simulink model "WiperSystemStateflow"  (R2022b)
settings: Solver=FixedStepDiscrete  StartTime=0.0  StopTime=20  FixedStep=0.01  RelTol=1e-3
undefined symbols (not defined in the file): sigbuilder_block
libraries: eeGeneralControl x1
settings Model: Creator=AymanLaptop  LastModifiedBy=AymanLaptop

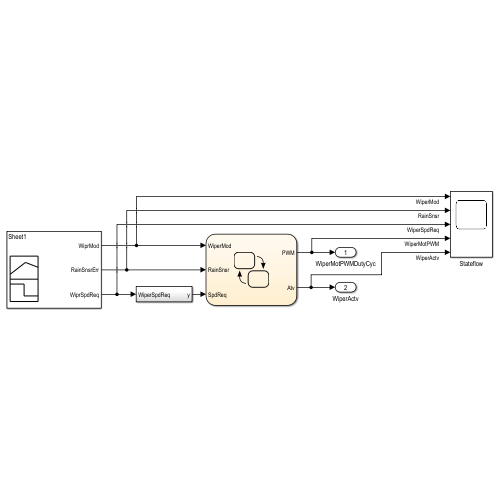
[thumbnail: Simulink's stored preview of the top-level diagram]
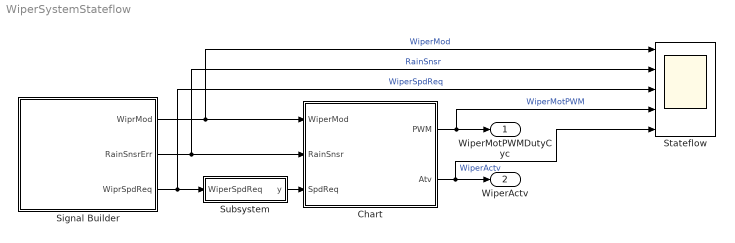
== system WiperSystemStateflow ==
  Chart : Stateflow chart  TreatAsAtomicUnit=on
      settings: PortSchema="{\"entries\":[{\"content\":{\"sides\":[{\"content\":{\"connectorIds\":[\"In2\",\"In1\",\"In3\"]},\"type\":\"ConnectorPlacement.EquallySpacedRectSide\",\"uuid\":\"e733ae65-f33e-49b0-845d-2dd686951ef3\"},{\"content\":{\"connectorIds\":[\"Out1\",\"Out2\"],\"side\":\"RIGHT\"},\"type\":\"ConnectorPlacement.EquallySpacedRectSide\",\"uuid\":\"70e09a91-b04b-4e75-a97f-4ab4b2922f79\"},{\"content\":{\"connectorIds\":[],\"side\":\"TOP\"},\"type\":\"ConnectorPlacement.EquallySpacedRectSide\",\"uuid\":\"7af5aa97-ae43-4f6a-8202-2e08a2f2b9b4\"}]},\"type\":\"ConnectorPlacement.EquallySpacedConnector\",\"uuid\":\"991bf9ea-0f6f-4566-8b19-b62aabc6abff\"}],\"packageUris\":[\"http://schema.mathworks.com/mf0/Connector/R2020b\"],\"version\":\"1.0\"}"
  Signal Builder : Subsystem  Tag=STV Subsys  LoadFcn=sigbuilder_block('load');  StartFcn=sigbuilder_block('start');  StopFcn=sigbuilder_block('stop');  ClipboardFcn=sigbuilder_block('clipboard');  mask(Sigbuilder block){tuvar=[0:10]}
      mask help: Simulink:masks:SigbuilderBlock_MD
      mask init:
      | if ~strcmp(get_param(bdroot(gcbh),'SimulationStatus'),'stopped') tuvar = sigbuilder_block('maskInit'); end
      settings: CopyFcn=sigbuilder_block('copy');  DeleteFcn=sigbuilder_block('delete');  ModelCloseFcn=sigbuilder_block('modelClose');  PreSaveFcn=sigbuilder_block('preSave');  PauseFcn=sigbuilder_block('pause');  ContinueFcn=sigbuilder_block('continue');  NameChangeFcn=sigbuilder_block('namechange');  OpenFcn=sigbuilder_block('open',[6 0 1012.5 455.25 ]);  CloseFcn=sigbuilder_block('close');
      mask Display: plot(0, 0, 100, 100,[2, 2, 32, 32, 2], [68, 8, 8, 68, 68],[32, 2], [38, 38], [32, 19, 2],[53, 60, 44], [32, 17, 17, 2],[16, 16, 31, 31]);txt = getActiveGroup(gcbh);text(2, 100, txt,'verticalAlignment', 'top');
  Stateflow : Scope  NumInputPorts=5
  Subsystem : Subsystem
  WiperMotPWMDutyCyc : Outport
  WiperActv : Outport  Port=2
  wires:
  Chart/2(Atv) -> WiperActv/1, Stateflow/5  "WiperActv"
  Signal Builder/1(WiprMod) -> Chart/2(WiperMod), Stateflow/1  "WiperMod"
  Signal Builder/3(WiprSpdReq) -> Stateflow/3, Subsystem/1(WiperSpdReq)  "WiperSpdReq"
  Signal Builder/2(RainSnsrErr) -> Chart/1(RainSnsr), Stateflow/2  "RainSnsr"
  Chart/1(PWM) -> WiperMotPWMDutyCyc/1, Stateflow/4  "WiperMotPWM"
  Subsystem/1(y) -> Chart/3(SpdReq)

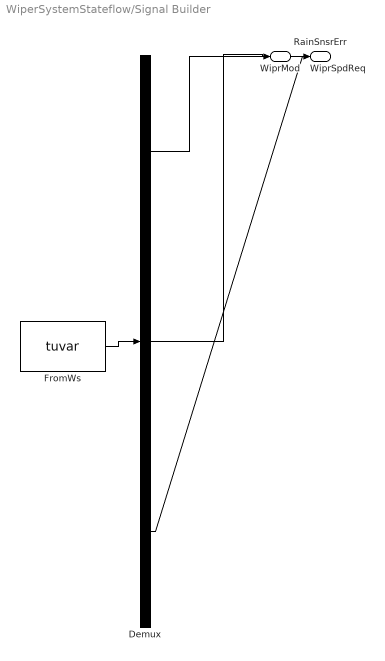
== system WiperSystemStateflow/Signal Builder ==
  Demux : Demux  Tag=STV Demux  Outputs=3
      settings: DisplayOption=none
  FromWs : FromWorkspace  Tag=STV FromWs  VariableName=tuvar  SampleTime=1  OutputAfterFinalValue=Holding final value
      SigBuilderData=|
      | common.afterFinalStr = 'Hold final value'
      | common.sampleTime = '1'
      | dataSet.timeRange = [0 16]
      | dataSet.name = 'Sheet1'
      | sbobj.Groups.Name = 'Sheet1'
      | sbobj.Groups.Signals(1).Name = 'WiprMod'
      | sbobj.Groups.Signals(1).XData = [0 1 2 3 4 5 6 7 8 9 10 11 12 13 14 15 16]
      | sbobj.Groups.Signals(1).YData = [0 0 2 2 3 3 1 1 1 1 1 1 1 1 1 1 1]
      | sbobj.Groups.Signals(2).Name = 'RainSnsrErr'
      | sbobj.Groups.Signals(2).XData = [0 1 2 3 4 5 6 7 8 9 10 11 12 13 14 15 16]
      | sbobj.Groups.Signals(2).YData = [0 0 0 0 0 0 0 0 0 0 0 0 0 0 0 1 0]
      | sbobj.Groups.Signals(3).Name = 'WiprSpdReq'
      | sbobj.Groups.Signals(3).XData = [0 1 2 3 4 5 6 7 8 9 10 11 12 13 14 15 16]
      | sbobj.Groups.Signals(3).YData = [0 0 0 0 0 0 0 0 1 2 3 4 5 6 7 7 7]
      | sbobj.Groups.TimeRange = [0 16]
  WiprMod : Outport  Tag=STV Outport
  RainSnsrErr : Outport  Tag=STV Outport  Port=2
  WiprSpdReq : Outport  Tag=STV Outport  Port=3
  wires:
  Demux/1 -> WiprMod/1
  FromWs/1 -> Demux/1
  Demux/2 -> RainSnsrErr/1
  Demux/3 -> WiprSpdReq/1

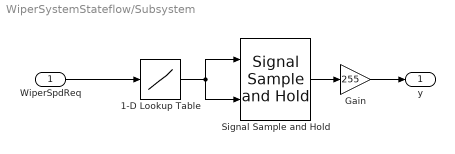
== system WiperSystemStateflow/Subsystem ==
  WiperSpdReq : Inport
  1-D Lookup Table : Lookup_n-D  NumberOfTableDimensions=1  BreakpointsForDimension1=[0 1 2 3 4 5 6 7]  Table=[0 0.40 0.45 0.50 0.55 0.60 0.65 0.70]  DiagnosticForOutOfRangeInput=Warning  RemoveProtectionInput=on  InternalRulePriority=Speed  RndMeth=Simplest
  Gain : Gain  Gain=255
  Signal Sample and Hold : eeGeneralControl/Signal Sample and Hold  LabelModeActiveChoice=Discrete  x0=0  Ts=-1
      settings: LibrarySourceBlock=ee_sl_lib/General Control/Signal Sample and Hold
  y : Outport
  wires:
  1-D Lookup Table/1 -> Signal Sample and Hold/1, Signal Sample and Hold/2
  WiperSpdReq/1 -> 1-D Lookup Table/1
  Signal Sample and Hold/1 -> Gain/1
  Gain/1 -> y/1

== stateflow chart WiperSystemStateflow/Chart ==
  state Off
    entry:
    PWM = 0;
    Atv = 0;
  state Auto
    entry, during:
    PWM = SpdReq;
    if PWM
    Atv = 1;
    else
    Atv = 0;
    end
  state High
    entry:
    PWM = 0.7*255;
    Atv = 1;
  state Low
    entry:
    PWM = 0.4*255;
    Atv = 1;
  (default) -> Off
  High -> Off [order 1] : [WiperMod == 0 || RainSnsr]
  Off -> High [order 2] : [WiperMod == 3 && ~RainSnsr]
  Auto -> Off [order 1] : [WiperMod == 0 || RainSnsr]
  Off -> Auto [order 1] : [WiperMod == 1 && ~RainSnsr]
  Low -> Off [order 1] : [WiperMod == 0 || RainSnsr]
  Off -> Low [order 3] : [WiperMod == 2 && ~RainSnsr]
  High -> Auto [order 2] : [WiperMod == 1]
  Low -> Auto [order 2] : [WiperMod == 1]
  Auto -> High [order 2] : [WiperMod == 3]
  Auto -> Low [order 3] : [WiperMod == 2]
  High -> Low [order 3] : [WiperMod == 2]
  Low -> High [order 3] : [WiperMod == 3]
  data: RainSnsr input; WiperMod input; PWM output; Atv output; SpdReq input
